simulink model "revision2"  (R2020a)
settings: Solver=VariableStepAuto  StartTime=0.0  StopTime=300  RelTol=1e-10
values from neighbouring files (symbols this model uses):
  a = 0.9897    [cal_z.m]    (also in simu.m)
  b = 0.05263    [cal_z.m]    (also in simu.m)
  d = 0    [cal_z.m]    (also in simu.m = 2)
  gamma = 0.1    [cal_z.m]    (also in simu.m)
  ki = 20    [simu.m]
  kp = 20    [simu.m]
libraries: simulink x3
settings Model: Creator=Lenovo  LastModifiedBy=Lenovo
settings SolverCC: ZeroCrossAlgorithm=Adaptive

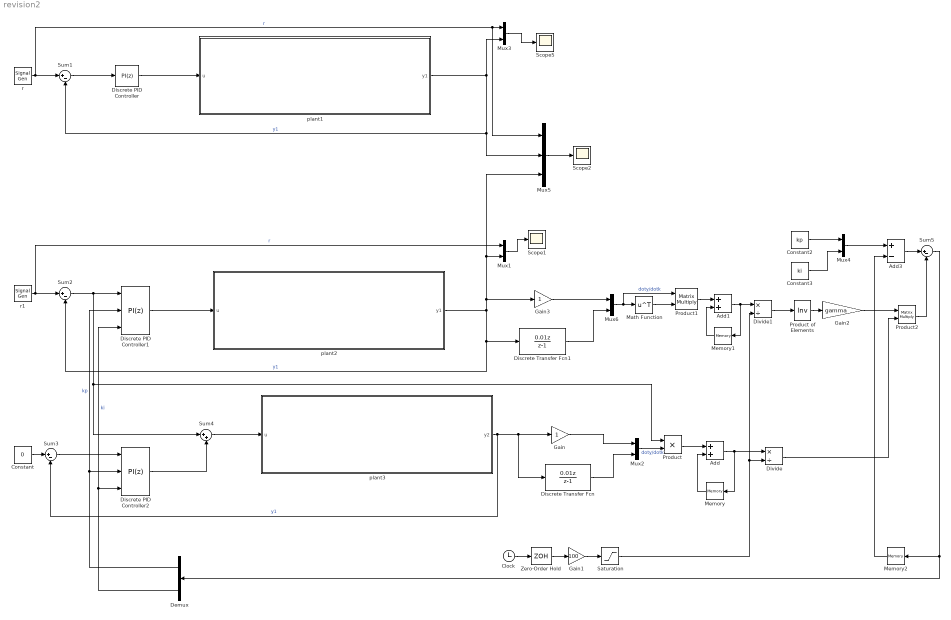
== system revision2 ==
  Add : Sum
  Add1 : Sum
  Add3 : Sum  Inputs=+-
  Clock : Clock
  Constant : Constant  Value=0  SampleTime=0.01
  Constant2 : Constant  Value=kp
  Constant3 : Constant  Value=ki
  Demux : Demux  Outputs=2
  Discrete Transfer Fcn : DiscreteTransferFcn  Numerator=[0.01 0]  Denominator=[1 -1]  SampleTime=0.01
  Discrete Transfer Fcn1 : DiscreteTransferFcn  Numerator=[0.01 0]  Denominator=[1 -1]  SampleTime=0.01
  Discrete PID Controller : simulink/Continuous/PID Controller  Controller=PI  Form=Parallel  TimeDomain=Discrete-time  UseExternalTs=off  SampleTime=0.01  IntegratorMethod=Forward Euler  FilterMethod=Forward Euler  ControllerParametersSource=internal  P=kp  I=ki  D=0  UseFilter=on  N=100  TunerSelectOption=Transfer Function Based (PID Tuner App)  InitialConditionSource=internal  InitialConditionForIntegrator=0  InitialConditionForFilter=0  DifferentiatorICPrevScaledInput=0  ExternalReset=none  TrackingMode=off  Kt=1  LimitOutput=off  UpperSaturationLimit=inf  LowerSaturationLimit=-inf  LinearizeAsGain=off  AntiWindupMode=none  Kb=1  POutMin=[]  POutMax=[]  IOutMin=[]  IOutMax=[]  DOutMin=[]  DOutMax=[]  NOutMin=[]  NOutMax=[]  SumOutMin=[]  SumOutMax=[]  SaturationOutMin=[]  SaturationOutMax=[]  PParamMin=[]  PParamMax=[]  IParamMin=[]  IParamMax=[]  DParamMin=[]  DParamMax=[]  NParamMin=[]  NParamMax=[]  KbParamMin=[]  KbParamMax=[]  KtParamMin=[]  KtParamMax=[]  KbOutMin=[]  KbOutMax=[]  KtOutMin=[]  KtOutMax=[]  IntegratorOutMin=[]  IntegratorOutMax=[]  FilterOutMin=[]  FilterOutMax=[]  SumI1OutMin=[]  SumI1OutMax=[]  SumI2OutMin=[]  SumI2OutMax=[]  SumI3OutMin=[]  SumI3OutMax=[]  SumI4OutMin=[]  SumI4OutMax=[]  SumDOutMin=[]  SumDOutMax=[]  DifferentiatorOutMin=[]  DifferentiatorOutMax=[]  FilterDiffOutCoefMin=[]  FilterDiffOutCoefMax=[]  ReciprocalOutMin=[]  ReciprocalOutMax=[]  SumDenOutMin=[]  SumDenOutMax=[]  SumNumOutMin=[]  SumNumOutMax=[]  DivideOutMin=[]  DivideOutMax=[]  UdiffTsProdOutMin=[]  UdiffTsProdOutMax=[]  NTsProdOutMin=[]  NTsProdOutMax=[]  UintegralTsProdOutMin=[]  UintegralTsProdOutMax=[]  UngainTsProdOutMin=[]  UngainTsProdOutMax=[]  IntegratorContinuousStateAttributes=''  IntegratorStateMustResolveToSignalObject=off  IntegratorRTWStateStorageClass=Auto  FilterContinuousStateAttributes=''  FilterStateMustResolveToSignalObject=off  FilterRTWStateStorageClass=Auto  ParallelPVariant=InternalParameters  IdealPVariant=Disabled  IVariant=InternalParameters  DVariant=Disabled  IntegratorVariant=Discrete  SatVariant=Disabled  AWVariant=Passthrough  PCopyVariant=Disabled  TRVariant=Disabled  FdbkBlocksVariant=Forward  IdealPFdbkVariant=Disabled  SatFdbkVariant=Disabled  DerivativeFilterVariant=Disabled  NVariant=Disabled  NCopyVariant=Disabled_SignalSpec  FilterICVariant=Disabled  IntegratorICVariant=InternalICs  ExternalResetVariant=Disabled  TRSumVariant=Passthrough  SumFdbkVariant=Disabled  SumVariant=Sum_PI  TsampFilterVariant=InternalTs  TsampNgainVariant=Passthrough  TsampIntegralVariant=Passthrough
  Discrete PID Controller1 : simulink/Continuous/PID Controller  Controller=PI  Form=Parallel  TimeDomain=Discrete-time  UseExternalTs=off  SampleTime=0.01  IntegratorMethod=Forward Euler  FilterMethod=Forward Euler  ControllerParametersSource=external  P=kp  I=ki  D=0  UseFilter=on  N=100  TunerSelectOption=Transfer Function Based (PID Tuner App)  InitialConditionSource=internal  InitialConditionForIntegrator=0  InitialConditionForFilter=0  DifferentiatorICPrevScaledInput=0  ExternalReset=none  TrackingMode=off  Kt=1  LimitOutput=off  UpperSaturationLimit=inf  LowerSaturationLimit=-inf  LinearizeAsGain=off  AntiWindupMode=none  Kb=1  POutMin=[]  POutMax=[]  IOutMin=[]  IOutMax=[]  DOutMin=[]  DOutMax=[]  NOutMin=[]  NOutMax=[]  SumOutMin=[]  SumOutMax=[]  SaturationOutMin=[]  SaturationOutMax=[]  PParamMin=[]  PParamMax=[]  IParamMin=[]  IParamMax=[]  DParamMin=[]  DParamMax=[]  NParamMin=[]  NParamMax=[]  KbParamMin=[]  KbParamMax=[]  KtParamMin=[]  KtParamMax=[]  KbOutMin=[]  KbOutMax=[]  KtOutMin=[]  KtOutMax=[]  IntegratorOutMin=[]  IntegratorOutMax=[]  FilterOutMin=[]  FilterOutMax=[]  SumI1OutMin=[]  SumI1OutMax=[]  SumI2OutMin=[]  SumI2OutMax=[]  SumI3OutMin=[]  SumI3OutMax=[]  SumI4OutMin=[]  SumI4OutMax=[]  SumDOutMin=[]  SumDOutMax=[]  DifferentiatorOutMin=[]  DifferentiatorOutMax=[]  FilterDiffOutCoefMin=[]  FilterDiffOutCoefMax=[]  ReciprocalOutMin=[]  ReciprocalOutMax=[]  SumDenOutMin=[]  SumDenOutMax=[]  SumNumOutMin=[]  SumNumOutMax=[]  DivideOutMin=[]  DivideOutMax=[]  UdiffTsProdOutMin=[]  UdiffTsProdOutMax=[]  NTsProdOutMin=[]  NTsProdOutMax=[]  UintegralTsProdOutMin=[]  UintegralTsProdOutMax=[]  UngainTsProdOutMin=[]  UngainTsProdOutMax=[]  IntegratorContinuousStateAttributes=''  IntegratorStateMustResolveToSignalObject=off  IntegratorRTWStateStorageClass=Auto  FilterContinuousStateAttributes=''  FilterStateMustResolveToSignalObject=off  FilterRTWStateStorageClass=Auto  ParallelPVariant=ExternalParameters  IdealPVariant=Disabled  IVariant=ExternalParameters  DVariant=Disabled  IntegratorVariant=Discrete  SatVariant=Disabled  AWVariant=Passthrough  PCopyVariant=Disabled  TRVariant=Disabled  FdbkBlocksVariant=Forward  IdealPFdbkVariant=Disabled  SatFdbkVariant=Disabled  DerivativeFilterVariant=Disabled  NVariant=Disabled  NCopyVariant=Disabled_SignalSpec  FilterICVariant=Disabled  IntegratorICVariant=InternalICs  ExternalResetVariant=Disabled  TRSumVariant=Passthrough  SumFdbkVariant=Disabled  SumVariant=Sum_PI  TsampFilterVariant=InternalTs  TsampNgainVariant=Passthrough  TsampIntegralVariant=Passthrough
  Discrete PID Controller2 : simulink/Continuous/PID Controller  Controller=PI  Form=Parallel  TimeDomain=Discrete-time  UseExternalTs=off  SampleTime=0.01  IntegratorMethod=Forward Euler  FilterMethod=Forward Euler  ControllerParametersSource=external  P=kp  I=ki  D=0  UseFilter=on  N=100  TunerSelectOption=Transfer Function Based (PID Tuner App)  InitialConditionSource=internal  InitialConditionForIntegrator=0  InitialConditionForFilter=0  DifferentiatorICPrevScaledInput=0  ExternalReset=none  TrackingMode=off  Kt=1  LimitOutput=off  UpperSaturationLimit=inf  LowerSaturationLimit=-inf  LinearizeAsGain=off  AntiWindupMode=none  Kb=1  POutMin=[]  POutMax=[]  IOutMin=[]  IOutMax=[]  DOutMin=[]  DOutMax=[]  NOutMin=[]  NOutMax=[]  SumOutMin=[]  SumOutMax=[]  SaturationOutMin=[]  SaturationOutMax=[]  PParamMin=[]  PParamMax=[]  IParamMin=[]  IParamMax=[]  DParamMin=[]  DParamMax=[]  NParamMin=[]  NParamMax=[]  KbParamMin=[]  KbParamMax=[]  KtParamMin=[]  KtParamMax=[]  KbOutMin=[]  KbOutMax=[]  KtOutMin=[]  KtOutMax=[]  IntegratorOutMin=[]  IntegratorOutMax=[]  FilterOutMin=[]  FilterOutMax=[]  SumI1OutMin=[]  SumI1OutMax=[]  SumI2OutMin=[]  SumI2OutMax=[]  SumI3OutMin=[]  SumI3OutMax=[]  SumI4OutMin=[]  SumI4OutMax=[]  SumDOutMin=[]  SumDOutMax=[]  DifferentiatorOutMin=[]  DifferentiatorOutMax=[]  FilterDiffOutCoefMin=[]  FilterDiffOutCoefMax=[]  ReciprocalOutMin=[]  ReciprocalOutMax=[]  SumDenOutMin=[]  SumDenOutMax=[]  SumNumOutMin=[]  SumNumOutMax=[]  DivideOutMin=[]  DivideOutMax=[]  UdiffTsProdOutMin=[]  UdiffTsProdOutMax=[]  NTsProdOutMin=[]  NTsProdOutMax=[]  UintegralTsProdOutMin=[]  UintegralTsProdOutMax=[]  UngainTsProdOutMin=[]  UngainTsProdOutMax=[]  IntegratorContinuousStateAttributes=''  IntegratorStateMustResolveToSignalObject=off  IntegratorRTWStateStorageClass=Auto  FilterContinuousStateAttributes=''  FilterStateMustResolveToSignalObject=off  FilterRTWStateStorageClass=Auto  ParallelPVariant=ExternalParameters  IdealPVariant=Disabled  IVariant=ExternalParameters  DVariant=Disabled  IntegratorVariant=Discrete  SatVariant=Disabled  AWVariant=Passthrough  PCopyVariant=Disabled  TRVariant=Disabled  FdbkBlocksVariant=Forward  IdealPFdbkVariant=Disabled  SatFdbkVariant=Disabled  DerivativeFilterVariant=Disabled  NVariant=Disabled  NCopyVariant=Disabled_SignalSpec  FilterICVariant=Disabled  IntegratorICVariant=InternalICs  ExternalResetVariant=Disabled  TRSumVariant=Passthrough  SumFdbkVariant=Disabled  SumVariant=Sum_PI  TsampFilterVariant=InternalTs  TsampNgainVariant=Passthrough  TsampIntegralVariant=Passthrough
  Divide : Product  Inputs=*/
  Divide1 : Product  Inputs=*/
  Gain : Gain
  Gain1 : Gain  Gain=100
  Gain2 : Gain  Gain=gamma
  Gain3 : Gain
  Math Function : Math  Operator=transpose  SaturateOnIntegerOverflow=on
  Memory : Memory  LinearizeAsDelay=on
  Memory1 : Memory  LinearizeAsDelay=on
  Memory2 : Memory  LinearizeAsDelay=on
  Mux{1..4,6} (5 alike) : Mux  Inputs=2
  Mux5 : Mux  Inputs=3
  Product : Product
  Product of Elements : Product  Inputs=/  Multiplication=Matrix(*)
  Product1 : Product  Multiplication=Matrix(*)
  Product2 : Product  Multiplication=Matrix(*)
  Saturation : Saturate  UpperLimit=inf  LowerLimit=1
  Scope1 : Scope
  Scope2 : Scope
  Scope5 : Scope
  Sum{1..3,5} (4 alike) : Sum  Inputs=|+-
  Sum4 : Sum  Inputs=|++
  Zero-Order Hold : ZeroOrderHold  SampleTime=0.01
  plant1 : Subsystem
  plant2 : Subsystem
  plant3 : Subsystem
  r : SignalGenerator  Frequency=0.001
  r1 : SignalGenerator  Frequency=0.001
  wires:
  Discrete PID Controller/1 -> plant1/1(u)
  Sum1/1 -> Discrete PID Controller/1
  r/1 -> Mux5/1, Mux3/1, Sum1/1  "r"
  plant1/1(y1) -> Mux3/2, Sum1/2, Mux5/2  "y1"
  Mux3/1 -> Scope5/1
  Discrete PID Controller1/1 -> plant2/1(u)
  Mux1/1 -> Scope1/1
  r1/1 -> Mux1/1, Sum2/1  "r"
  Sum2/1 -> Product/1, Sum4/1, Discrete PID Controller1/1
  Constant/1 -> Sum3/1
  Sum3/1 -> Discrete PID Controller2/1
  Discrete PID Controller2/1 -> Sum4/2
  Sum4/1 -> plant3/1(u)
  Gain/1 -> Mux2/1
  Discrete Transfer Fcn/1 -> Mux2/2
  plant3/1(y2) -> Gain/1, Discrete Transfer Fcn/1, Sum3/2  "y1"
  Mux2/1 -> Product/2  "doty/dotk"
  Add/1 -> Memory/1, Divide/1
  Gain1/1 -> Saturation/1
  Clock/1 -> Zero-Order Hold/1
  Memory/1 -> Add/2
  Zero-Order Hold/1 -> Gain1/1
  Product/1 -> Add/1
  Product1/1 -> Add1/1
  Product of Elements/1 -> Gain2/1
  Divide1/1 -> Product of Elements/1
  Add1/1 -> Divide1/1, Memory1/1
  Memory1/1 -> Add1/2
  Math Function/1 -> Product1/2
  Saturation/1 -> Divide1/2, Divide/2
  Gain2/1 -> Product2/1
  Mux4/1 -> Add3/1
  Add3/1 -> Sum5/1
  Product2/1 -> Sum5/2
  Memory2/1 -> Add3/2
  Constant2/1 -> Mux4/1
  Constant3/1 -> Mux4/2
  Divide/1 -> Product2/2
  Demux/1 -> Discrete PID Controller1/2, Discrete PID Controller2/2  "kp"
  Demux/2 -> Discrete PID Controller1/3, Discrete PID Controller2/3  "ki"
  Sum5/1 -> Demux/1, Memory2/1
  Mux5/1 -> Scope2/1
  Gain3/1 -> Mux6/1
  plant2/1(y1) -> Gain3/1, Mux5/3, Mux1/2, Discrete Transfer Fcn1/1, Sum2/2  "y1"
  Discrete Transfer Fcn1/1 -> Mux6/2
  Mux6/1 -> Product1/1, Math Function/1  "doty/dotk"

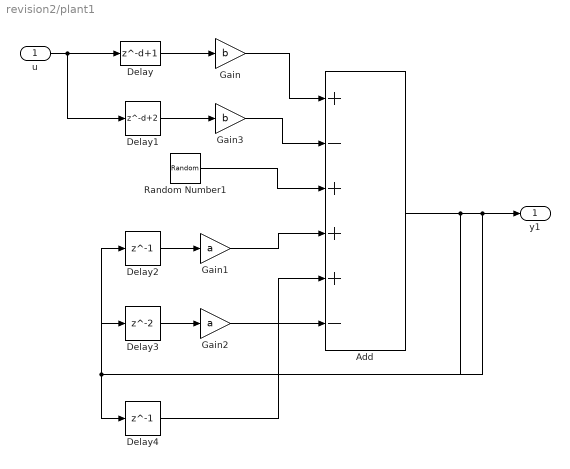
== system revision2/plant1 ==
  u : Inport
  Add : Sum  Inputs=+-+++-
  Delay : Delay  DelayLength=d+1  InitialCondition=0  SampleTime=0.01
  Delay1 : Delay  DelayLength=d+2  InitialCondition=0  SampleTime=0.01
  Delay2 : Delay  DelayLength=1  InitialCondition=0  SampleTime=0.01
  Delay3 : Delay  InitialCondition=0  SampleTime=0.01
  Delay4 : Delay  DelayLength=1  InitialCondition=0  SampleTime=0.01
  Gain : Gain  Gain=b
  Gain1 : Gain  Gain=a
  Gain2 : Gain  Gain=a
  Gain3 : Gain  Gain=b
  Random Number1 : RandomNumber  Variance=0.0000001  SampleTime=0.01
  y1 : Outport
  wires:
  Delay/1 -> Gain/1
  u/1 -> Delay1/1, Delay/1
  Delay1/1 -> Gain3/1
  Gain/1 -> Add/1
  Gain3/1 -> Add/2
  Random Number1/1 -> Add/3
  Delay2/1 -> Gain1/1
  Delay3/1 -> Gain2/1
  Add/1 -> Delay4/1, Delay2/1, Delay3/1, y1/1
  Gain1/1 -> Add/4
  Gain2/1 -> Add/6
  Delay4/1 -> Add/5

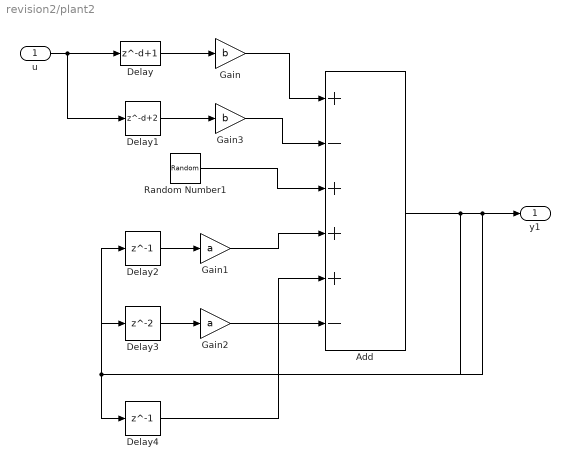
== system revision2/plant2 ==
  u : Inport
  Add : Sum  Inputs=+-+++-
  Delay : Delay  DelayLength=d+1  InitialCondition=0  SampleTime=0.01
  Delay1 : Delay  DelayLength=d+2  InitialCondition=0  SampleTime=0.01
  Delay2 : Delay  DelayLength=1  InitialCondition=0  SampleTime=0.01
  Delay3 : Delay  InitialCondition=0  SampleTime=0.01
  Delay4 : Delay  DelayLength=1  InitialCondition=0  SampleTime=0.01
  Gain : Gain  Gain=b
  Gain1 : Gain  Gain=a
  Gain2 : Gain  Gain=a
  Gain3 : Gain  Gain=b
  Random Number1 : RandomNumber  Variance=0.0000001  SampleTime=0.01
  y1 : Outport
  wires:
  Delay/1 -> Gain/1
  u/1 -> Delay1/1, Delay/1
  Delay1/1 -> Gain3/1
  Gain/1 -> Add/1
  Gain3/1 -> Add/2
  Random Number1/1 -> Add/3
  Delay2/1 -> Gain1/1
  Delay3/1 -> Gain2/1
  Add/1 -> Delay4/1, Delay2/1, Delay3/1, y1/1
  Gain1/1 -> Add/4
  Gain2/1 -> Add/6
  Delay4/1 -> Add/5

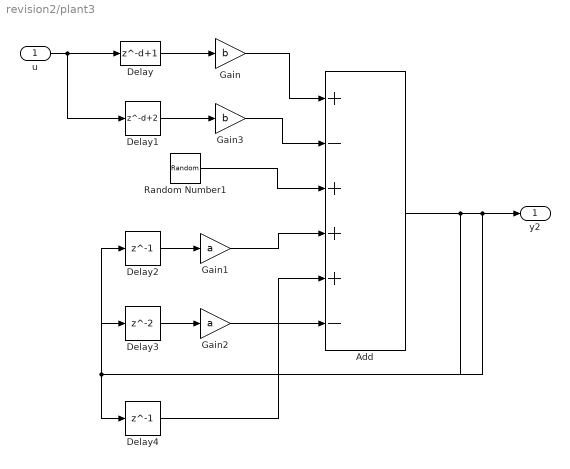
== system revision2/plant3 ==
  u : Inport
  Add : Sum  Inputs=+-+++-
  Delay : Delay  DelayLength=d+1  InitialCondition=0  SampleTime=0.01
  Delay1 : Delay  DelayLength=d+2  InitialCondition=0  SampleTime=0.01
  Delay2 : Delay  DelayLength=1  InitialCondition=0  SampleTime=0.01
  Delay3 : Delay  InitialCondition=0  SampleTime=0.01
  Delay4 : Delay  DelayLength=1  InitialCondition=0  SampleTime=0.01
  Gain : Gain  Gain=b
  Gain1 : Gain  Gain=a
  Gain2 : Gain  Gain=a
  Gain3 : Gain  Gain=b
  Random Number1 : RandomNumber  Variance=0.0000001  SampleTime=0.01
  y2 : Outport
  wires:
  Delay/1 -> Gain/1
  u/1 -> Delay1/1, Delay/1
  Delay1/1 -> Gain3/1
  Gain/1 -> Add/1
  Gain3/1 -> Add/2
  Random Number1/1 -> Add/3
  Delay2/1 -> Gain1/1
  Delay3/1 -> Gain2/1
  Add/1 -> Delay4/1, Delay2/1, Delay3/1, y2/1
  Gain1/1 -> Add/4
  Gain2/1 -> Add/6
  Delay4/1 -> Add/5
